simulink library "embdlinuxlib"  (R2018b)
settings: Solver=ode45  StartTime=0.0  StopTime=10.0  RelTol=1e-3
undefined symbols (not defined in the file or in its folder): gcbh, hw, realtime
settings Model: FPTRunName=Active  ModifiedByFormat=The MathWorks Inc.  Creator=The MathWorks, Inc.  LastModifiedBy=The MathWorks Inc.
settings DataIOCC: LimitDataPoints=on  SaveFormat=Array  SignalLoggingSaveFormat=ModelDataLogs
settings OptimizationCC: BlockReduction=off  BooleanDataType=off  ExpressionDepthLimit=2147483647  LifeSpan=inf
settings DebuggingCC: SaveWithParameterizedLinksMsg=none  UnderspecifiedInitializationDetection=Classic  MergeDetectMultiDrivingBlocksExec=none  SignalResolutionControl=TryResolveAllWithWarning  FcnCallInpInsideContextMsg=warning  AllowSymbolicDim=off  StateNameClashWarn=warning  LibraryContextMissingDiagnostic=none  SFUnexpectedBacktrackingDiag=warning  SFNoUnconditionalDefaultTransitionDiag=warning  SFExecutionAtInitializationDiag=none
settings HardwareCC: ProdBitPerPointer=32  ProdBitPerSizeT=32  ProdBitPerPtrDiffT=32  ProdLargestAtomicFloat=None  ProdIntDivRoundTo=Undefined  ProdEndianess=Unspecified  ProdWordSize=32  ProdHWDeviceType=32-bit Generic  TargetUnknown=on
settings ModelReferenceCC: PropagateSignalLabelsOutOfModel=off
settings SFSimCC: SimUseLocalCustomCode=off
settings RTWCC: RTWUseLocalCustomCode=off
settings CodeAppCC: StateflowObjectComments=on
settings GRTTargetCC: TargetLangStandard=C89/C90 (ANSI)  GeneratePreprocessorConditionals=Disable all  CombineOutputUpdateFcns=off  GRTInterface=on
settings ConfigComp: CovMetricSettings=dw  CovHtmlReporting=on  CovSaveCumulativeToWorkspaceVar=on  CovSaveSingleToWorkspaceVar=on  CovShowResultsExplorer=off  CovExternalEMLEnable=off  CovSFcnEnable=off

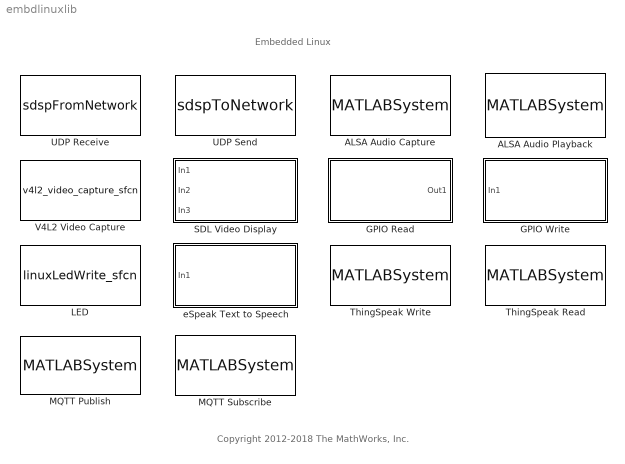
== system embdlinuxlib ==
  note: Copyright 2012-2018 The MathWorks, Inc.
  note: Embedded Linux
  ALSA Audio Capture : MATLABSystem  InitFcn=realtime.internal.ALSAAudioCaptureCallback(gcbh)  System=codertarget.linux.blocks.ALSAAudioCapture  deviceStr=hw:1,0  DataBitDepth=16-bit integer  numberOfChannels=numberOfChannels  sampleRateEnum=sampleRateEnum  frameSize=frameSize  QueueDuration=QueueDuration  blockPlatform=RASPBERRYPI  mask(codertarget.linux.blocks.ALSAAudioCapture){deviceStr=hw:1,0, DataBitDepth=16-bit integer, numberOfChannels=2, sampleRateEnum=44100, frameSize=4410, QueueDuration=0.5, blockPlatform=RASPBERRYPI}
      mask prompts: deviceStr "Device name:"; DataBitDepth "Device Bit depth:"; numberOfChannels "Number of channels(C):"; sampleRateEnum "Audio sampling frequency (Hz):"; frameSize "Samples per frame(N):"; QueueDuration "Queue duration (seconds):"; blockPlatform "Block platform:"
      mask help:
      | Captures audio from the sound card using ALSA driver framework.
      |
      | The block outputs audio data as NxC array, where N is the samples per audio channel and C is the number of chanels.
      |
      | Enter the device name and the number of channels supported by the device. Use the Audio sampling frequency parameter to set the sampling rate in Hertz(Hz). Sample time of the block will be derived from the sampling frequency and the Samples per frame(N) specified by the user.
      mask TypeOptions deviceStr: deviceStr
      mask TypeOptions DataBitDepth: DataBitDepth
      mask TypeOptions numberOfChannels: numberOfChannels
      mask TypeOptions sampleRateEnum: sampleRateEnum
      mask TypeOptions frameSize: frameSize
      mask TypeOptions QueueDuration: QueueDuration
      mask TypeOptions blockPlatform: blockPlatform
      mask Display:
      | color('white');
      | 
      | plot([100,100,100,100],[100,100,100,100]);
      | 
      | plot([0,0,0,0],[0,0,0,0]);
      | 
      | color('black');
      | 
      | text(50, 12,'Device: hw:1,0', 'horizontalAlignment','center','verticalAlignment','middle');
      | 
      | color('blue');
      | 
      | text(96, 90, 'RASPBERRYPI', 'horizontalAlignment', 'right');
      | 
      | color('black');
      | 
      | image('sound_sensor.gif','center');
  ALSA Audio Playback : MATLABSystem  System=codertarget.linux.blocks.ALSAAudioPlayback  deviceStr=hw:0,0  sampleRateEnum=sampleRateEnum  queueDuration=queueDuration  blockPlatform=RASPBERRYPI  mask(codertarget.linux.blocks.ALSAAudioPlayback){deviceStr=hw:0,0, sampleRateEnum=44100, queueDuration=0.5, blockPlatform=RASPBERRYPI}
      mask prompts: deviceStr "Device name:"; sampleRateEnum "Audio sampling frequency (Hz):"; queueDuration "Queue duration (seconds):"; blockPlatform "Block platform:"
      mask help:
      | Sends audio to the sound card for playback using ALSA driver framework.
      |
      | The block accepts NxC array of type int8, int16 or int32, where N is the samples per audio channel and C is the number of channels.
      |
      | Enter the device name and use the Audio sampling frequency parameter to set the sampling rate in Hertz (Hz).
      mask TypeOptions deviceStr: deviceStr
      mask TypeOptions sampleRateEnum: sampleRateEnum
      mask TypeOptions queueDuration: queueDuration
      mask TypeOptions blockPlatform: blockPlatform
      mask Display:
      | color('white');
      | 
      | plot([100,100,100,100],[100,100,100,100]);
      | 
      | plot([0,0,0,0],[0,0,0,0]);
      | 
      | color('black');
      | 
      | text(50, 12,'Device: hw:0,0', 'horizontalAlignment','center','verticalAlignment','middle');
      | 
      | color('blue');
      | 
      | text(96, 90, 'RASPBERRYPI', 'horizontalAlignment', 'right');
      | 
      | color('black');
      | 
      | image('speaker.gif','center');
  GPIO Read : Subsystem  DialogController=linuxDDGCreate  InitFcn=|  mask(GPIO Read){board=Model B+, gpio=17, internalResistor=Off, sampleTime=0.1, direction=Input, blockPlatform=Raspberry Pi}
      | realtime.internal.validateLinuxBlock(get_param(gcbh,'blockPlatform'), gcbh);
      | realtime.internal.gpioCheckParameters(gcs,gcb);
      | realtime.internal.validateGPIO(gcb);
      mask prompts: gpio "GPIO number:"; internalResistor "Internal resistor:"; sampleTime "Sample time:"; blockPlatform "Block platform:"
      mask help: Reads the logical value of a specified GPIO pin configured as input. Select the GPIO input number. Select the internal resistor. Use only one block per GPIO.
      mask init:
      | h = realtime.internal.BoardInfo(blockPlatform);
      | pinName = h.getGPIOPrimaryFunction(board, gpio);
      | pinName = uint8([pinName, 0]); % Add C string termination character
      | switch (internalResistor)
      |     case {'Off'}
      |         resistor = 1;
      |     case {'Pull-up'}
      |         resistor = 2;
      |     case {'Pull-down'}
      |         resistor = 3;
      |     otherwise
      |         resistor = 255; %N/A
      | end
      | realtime.internal.linuxGpioRead('MaskInitialization');
      mask Help: eval('realtime.helpView(get_param(gcb, ''blockPlatform''), [realtime.internal.getHelpLinkPrefix(gcb) ''libgpioread''])');
      mask TypeOptions direction: Input | Output
      mask Display:
      | text(0.5, 0.15, 'GPIO 17', 'horizontalAlignment', 'center');
      | image(imread('digitalio.png'),[0.32 0.25 0.35 0.55]);
      | color('blue');
      | text(0.90, 0.90, 'RASPBERRYPI', 'horizontalAlignment', 'right');
      | color('black');
  GPIO Write : Subsystem  DialogController=linuxDDGCreate  InitFcn=|  mask(GPIO Write){board=Model B+, gpio=4, direction=Output, blockPlatform=Raspberry Pi}
      | realtime.internal.validateLinuxBlock(get_param(gcbh,'blockPlatform'), gcbh);
      | realtime.internal.gpioCheckParameters(gcs,gcb);
      | realtime.internal.validateGPIO(gcb);
      mask prompts: gpio "GPIO number:"; blockPlatform "Block platform:"
      mask help: Sets the logical value of a GPIO pin configured as output. Select the GPIO output number. Do not assign the same GPIO number to multiple blocks within a model.
      mask init:
      | h = realtime.internal.BoardInfo(blockPlatform);
      | realtime.internal.linuxGpioWrite('MaskInitialization');
      mask Help: eval('realtime.helpView(get_param(gcb, ''blockPlatform''), [realtime.internal.getHelpLinkPrefix(gcb) ''libgpiowrite''])');
      mask TypeOptions direction: Input | Output
      mask Display:
      | text(0.5, 0.15, 'GPIO 4', 'horizontalAlignment', 'center');
      | image(imread('digitalio.png'),[0.32 0.25 0.35 0.55]);
      | color('blue');
      | text(0.90, 0.90, 'RASPBERRYPI', 'horizontalAlignment', 'right');
      | color('black');
  LED : S-Function  DialogController=linuxDDGCreate  InitFcn=realtime.internal.validateLinuxBlock(get_param(gcbh, 'blockPlatform'), gcbh);  FunctionName=linuxLedWrite_sfcn  Parameters=deviceFile  SFunctionDeploymentMode=off  EnableBusSupport=off  mask(LED Write){board=BeagleBoard xM, led=PMU_STAT (Green), blockPlatform=Raspberry Pi}
      mask prompts: blockPlatform "Block platform:"
      mask help:
      | Turns an LED on or off.
      |
      | Select the desired LED from the drop down menu. Do not use the same LED
      | in multiple blocks within a model.
      mask init:
      | hBoard = realtime.internal.BoardInfo(blockPlatform);
      | deviceFile = hBoard.getLEDDeviceFile(board, led);
      | deviceFile = uint8([deviceFile, 0]);
      | realtime.internal.linuxLedWrite('MaskInitialization');
      mask Help: eval('realtime.helpView(get_param(gcb, ''blockPlatform''),[realtime.internal.getHelpLinkPrefix(gcb) ''libled''])');
      mask Display:
      | text(0.5, 0.15, 'PMU_STAT (Green)', 'horizontalAlignment', 'center');
      | image(imread('led.png'),[0.32 0.25 0.35 0.55]);
      | color('blue');
      | text(0.90, 0.90, 'RASPBERRYPI', 'horizontalAlignment', 'right');
      | color('black');
  MQTT Publish : MATLABSystem  System=codertarget.linux.blocks.MQTTPublish  Topic=topic/level  QoS=0  RetainMsg=off
      mask Type: codertarget.linux.blocks.MQTTPublish
      mask Display:
      | color('white');
      | 
      | plot([100,100,100,100],[100,100,100,100]);
      | 
      | plot([0,0,0,0],[0,0,0,0]);
      | 
      | color('black');
      | 
      | port_label('input',1,'Msg');
      | 
      | port_label('output',1,'Status');
      | 
      | text(50, 12,'topic/level', 'horizontalAlignment','center','verticalAlignment','middle');
      | 
      | color('blue');
      | 
      | text(96, 90, 'RASPBERRYPI', 'horizontalAlignment', 'right');
  MQTT Subscribe : MATLABSystem  System=codertarget.linux.blocks.MQTTSubscribe  Topic=topic/level/#  QoS=0  MessageLength=1  SampleTime=1
      mask Type: codertarget.linux.blocks.MQTTSubscribe
      mask Display:
      | color('white');
      | 
      | plot([100,100,100,100],[100,100,100,100]);
      | 
      | plot([0,0,0,0],[0,0,0,0]);
      | 
      | color('black');
      | 
      | port_label('output',1,'IsNew');
      | 
      | port_label('output',3,'Topic');
      | 
      | port_label('output',2,'Msg');
      | 
      | text(50, 12,'topic/level/#', 'horizontalAlignment','center','verticalAlignment','middle');
      | 
      | color('blue');
      | 
      | text(96, 90, 'RASPBERRYPI', 'horizontalAlignment', 'right');
      | 
      | color('black');
  SDL Video Display : Subsystem  InitFcn=|  TreatAsAtomicUnit=on  mask(SDL Video Display){pixelFormat=RGB, pixelOrder=Planar, rowMajor=on, blockPlatform=Raspberry Pi}
      | realtime.internal.validateLinuxBlock(get_param(gcbh,'blockPlatform'),gcbh);
      | realtime.internal.sdl_video_display_callback('BlockCheck',gcbh);
      mask prompts: pixelFormat "Pixel format:"; pixelOrder "Pixel order:"; rowMajor "Input image is transposed (data is row major)"; blockPlatform "Block platform:"
      mask help: Displays video using Simple Directmedia Layer (SDL) multimedia library. Use Pixel format parameter to specify the format of the input video stream. Only one SDL Video Display block is allowed in a Simulink model.
      mask init:
      | realtime.internal.sdl_video_display_callback('MaskInitialization',gcbh);
      mask Help: eval('realtime.helpView(get_param(gcb, ''blockPlatform''),[realtime.internal.getHelpLinkPrefix(gcb) ''libsdlvideodisplay''])');
      mask TypeOptions pixelFormat: RGB | YCbCr 4:2:2
      mask TypeOptions pixelOrder: Planar | Interleaved
      mask Display:
      | color('blue');
      | text(0.90, 0.90, 'RASPBERRYPI', 'horizontalAlignment', 'right');
      | color('black');
      | [data, map]=imread('LCD.gif');pic=ind2rgb(data,map);image(pic,[0.32 0.25 0.35 0.55]);
      | port_label('input', 1, 'R');
      | port_label('input', 2, 'G');
      | port_label('input', 3, 'B');
  ThingSpeak Read : MATLABSystem  System=codertarget.linux.blocks.ThingSpeakRead  ChannelID=12345  ChannelAccess=Public  ReadAPIKey=ABCDEFGHIJK  FieldNumber=1  PrintDiagnosticMessages=off  SampleTime=60
      mask Type: codertarget.linux.blocks.ThingSpeakRead
      mask Display:
      | color('white');
      | 
      | plot([100,100,100,100],[100,100,100,100]);
      | 
      | plot([0,0,0,0],[0,0,0,0]);
      | 
      | color('black');
      | 
      | port_label('output',1,'Field1');
      | 
      | port_label('output',2,'Status');
      | 
      | text(50, 12,'Channel:12345', 'horizontalAlignment','center','verticalAlignment','middle');
      | 
      | color('blue');
      | 
      | text(96, 90, 'RASPBERRYPI', 'horizontalAlignment', 'right');
      | 
      | color('black');
      | 
      | image('cloudread_linux.png','center');
  ThingSpeak Write : MATLABSystem  InitFcn=realtime.internal.validateLinuxBlock(get_param(gcbh, 'blockPlatform'), gcbh);  System=codertarget.linux.blocks.ThingSpeakWrite  UpdateURL=https://api.thingspeak.com/update  WriteAPIKey=<Enter the write API key for your channel>  NumberOfVariables=1  UpdateInterval=UpdateInterval  PrintDiagnosticMessages=off  CoordinatesEnabled=off  CoordinatesSource=Block dialog  Coordinates=Coordinates  StatusEnabled=off  StatusSource=Block dialog  StatusMessage=OK  mask(codertarget.linux.blocks.ThingSpeakWrite){UpdateURL=https://api.thingspeak.com/update, WriteAPIKey=<Enter the write API key for your channel>, NumberOfFields=1, UpdateInterval=60, PrintDiagnosticMessages=off, CoordinatesEnabled=off, CoordSrc=Block dialog, Coordinates=[42.29971, -71.350719, 69.29], blockPlatform=Raspberry Pi}
      mask prompts: UpdateURL "Update URL:"; WriteAPIKey "Write API key:"; NumberOfFields "Number of variables to send:"; UpdateInterval "Update interval:"; PrintDiagnosticMessages "Print diagnostic messages"; CoordinatesEnabled "Send location information"; CoordSrc "Coordinate source:"; Coordinates "Coordinates (latitude, longitude, altitude):"; blockPlatform "Block platform:"
      mask help:
      | Send data to ThingSpeak, MathWorks IoT Analytics Platform.
      | The hardware must be connected to the Internet. Input ports only accept numeric scalar signals.
      |
      | Enter the Write API Key for your ThingSpeak channel. Each input variable is written to a field in your ThingSpeak channel.
      | Set Update interval to the number of seconds to wait between two successive data send requests. Visit your ThingSpeak account page to find the minimum update interval for your channel.
      |
      | Check “Print diagnostic messages” to send the ThingSpeak server response to standard output on the hardware.
      mask init:
      | codertarget.linux.blocks.ThingSpeakWriteCallback('MaskInitialization',gcbh);
      mask Help: eval('realtime.helpView(get_param(gcb, ''blockPlatform''), [realtime.internal.getHelpLinkPrefix(gcb) ''libthingspeakwrite''])');
      mask TypeOptions UpdateURL: UpdateURL
      mask TypeOptions WriteAPIKey: WriteAPIKey
      mask TypeOptions NumberOfFields: 1 | 2 | 3 | 4 | 5 | 6 | 7 | 8
      mask TypeOptions UpdateInterval: UpdateInterval
      mask TypeOptions PrintDiagnosticMessages: PrintDiagnosticMessages
      mask TypeOptions CoordinatesEnabled: CoordinatesEnabled
      mask Callback CoordinatesEnabled: codertarget.linux.blocks.ThingSpeakWriteCallback('CoordinatesEnabled',gcbh);
      mask TypeOptions CoordSrc: Block dialog | Input port
      mask Callback CoordSrc: codertarget.linux.blocks.ThingSpeakWriteCallback('CoordinatesSource',gcbh);
      mask TypeOptions Coordinates: Coordinates
      mask DialogControl DescGroupVar Prompt: ThingSpeak Write
      mask DialogControl Container2 Prompt: Main
      mask DialogControl Container10 Prompt: Optional
      mask Display:
      | image(imread('cloud.png'),[0.25 0.25 0.55 0.45]);
      | color('blue');
      | text(0.35, 0.87, 'RASPBERRYPI', 'horizontalAlignment', 'left');
      | color('black');
      | CoordinatesEnabled = get_param(gcb, 'CoordinatesEnabled');
      | CoordinatesSource = get_param(gcb, 'CoordinatesSource');
      | NumberOfFields_ = str2double(get_param(gcb,'NumberOfFields'));
      | if NumberOfFields_ >= 2
      | port_label('input', 1, 'var1');
      | port_label('input', 2, 'var2');
      | end
      | if NumberOfFields_ >= 3
      | port_label('input', 3, 'var3');
      | end
      | if NumberOfFields_ >= 4
      | port_label('input', 4, 'var4');
      | end
      | if NumberOfFields_ >= 5
      | port_label('input', 5, 'var5');
      | end
      | if NumberOfFields_ >= 6
      | port_label('input', 6, 'var6');
      | end
      | if NumberOfFields_ >= 7
      | port_label('input', 7, 'var7');
      | end
      | if NumberOfFields_ >= 8
      | port_label('input', 8, 'var8');
      | end
      | if strcmp(CoordinatesEnabled, 'on') && strcmp(CoordinatesSource, 'Input port')
      | port_label('input', NumberOfFields_+1, 'location');
      | end
  UDP Receive : S-Function  InitFcn=realtime.internal.validateLinuxBlock(get_param(gcbh, 'blockPlatform'), gcbh);  FunctionName=sdspFromNetwork  Parameters=localURL, localPort, remoteURL, remotePort, recvBufferSize, signalDatatype, dims, sampletime, isVarSize, blockingTime  SFunctionDeploymentMode=off  EnableBusSupport=off  mask(UDP Receive){localURL='0.0.0.0', localPort=25000, remoteURL='0.0.0.0', remotePort=-1, recvBufferSize=8192, signalDatatype=uint8, dims=255, isVarSize=off, showBlockingTime=off, blockingTime=0, sampletime=0.01, blockPlatform=Raspberry Pi}
      mask prompts: localURL "Local IP address:"; localPort "Local IP port:"; remoteURL "Remote IP address ('0.0.0.0' to accept all):"; remotePort "Remote IP port:"; recvBufferSize "Receive buffer size (bytes):"; signalDatatype "Data type:"; dims "Data size (elements):"; isVarSize "Output variable-size signal"; showBlockingTime "Show blocking time"; blockingTime "Blocking time (seconds):"; sampletime "Sample time (seconds):"; blockPlatform "Block Platform"
      mask help:
      | Receives UDP packets from another UDP host on an Internet network. The sending UDP host must send UDP packets to the Local IP port specified in the block mask.
      |
      | Match the Data type parameter with the data type of the incoming data. Match the Data size parameter with the number of elements of the incoming data.
      |
      | For example, if the data type of the incoming data is single and the dimensions are [3x1], set the Data type parameter to single and set the Data size parameter to 3.
      mask init:
      | icon = '';
      | %icon = sprintf('%s\n', 'fprintf(''UDP Receive'');');
      | % If there are multiple ports, label them
      | if strcmp(get_param(gcb,'isVarSize'), 'off')
      |     icon = sprintf('%s%s\n', icon, 'port_label(''output'', 1, ''Data'');');
      |     icon = sprintf('%s%s\n', icon, 'port_label(''output'', 2, ''Size'');');
      | end
      | icon = [icon sprintf('%s\n','color(''blue'');')];
      | icon = [icon '[data, map]=imread(''ethernet1_bw.gif'');pic=ind2rgb(data,map);image(pic,[0.32 0.25 0.40 0.45]);'];
      | platform = realtime.internal.getBlockDisplayText(gcb);
      | icon = [icon sprintf('%s\n',['text(0.97, 0.87, ''' platform ''', ''horizontalalignment'', ''right'');'])];
      | set_param(gcb, 'maskDisplay', icon);
      | 
      | % Hide the lengthDatatype and BlockingTime if required
      | vis = get_param(gcbh, 'MaskVisibilities');
      | vis{10} = get_param(gcbh, 'showBlockingTime');
      | set_param(gcbh, 'MaskVisibilities', vis);
      mask Help: eval('realtime.helpView(get_param(gcb, ''blockPlatform''), [realtime.internal.getHelpLinkPrefix(gcb) ''libudpreceive''])');
      mask TypeOptions signalDatatype: double | single | int8 | uint8 | int16 | uint16 | int32 | uint32 | boolean
      mask Display:
      | port_label('output', 1, 'Data');
      | port_label('output', 2, 'Size');
      | color('blue');
      | [data, map]=imread('ethernet1_bw.gif');pic=ind2rgb(data,map);image(pic,[0.32 0.25 0.40 0.45]);text(0.97, 0.87, 'RASPBERRYPI', 'horizontalalignment', 'right');
  UDP Send : S-Function  InitFcn=realtime.internal.validateLinuxBlock(get_param(gcbh, 'blockPlatform'), gcbh);  FunctionName=sdspToNetwork  Parameters=localURL, localPortSource, localPort, remoteURL, remotePort, separateLengthPort, []  SFunctionDeploymentMode=off  EnableBusSupport=off  mask(UDP Send){remoteURL='255.255.255.255', remotePort=25000, localURL='0.0.0.0', localPortSource=Automatically determine, localPort=-1, sampletime=-1, blockPlatform=Raspberry Pi, separateLengthPort=0}
      mask prompts: remoteURL "Remote IP address ('255.255.255.255' for broadcast):"; remotePort "Remote IP port:"; localURL "Local IP address:"; localPortSource "Local IP port source:"; localPort "Local IP port:"; blockPlatform "Block Platform"; separateLengthPort "Use a separate length port"
      mask help: Sends UDP packets to another UDP host on an Internet network. Set Remote IP address parameter to the IP address of the receiving UDP host. Set the Remote IP port parameter to the port number used by the receiving UDP host.
      mask Help: eval('realtime.helpView(get_param(gcb, ''blockPlatform''), [realtime.internal.getHelpLinkPrefix(gcb) ''libudpsend''])');
      mask TypeOptions localPortSource: Automatically determine | Specify via dialog
      mask Callback localPortSource:
      | mask_vis = get_param(gcbh, 'MaskVisibilities');
      | if strcmp(get_param(gcbh,'localPortSource'),'Specify via dialog')
      |     mask_vis{5} = 'on';
      | else
      |     mask_vis{5} = 'off';
      | end
      | set_param(gcbh, 'MaskVisibilities', mask_vis);
      | clear('mask_vis');
      mask Display:
      | %fprintf('UDP Send');
      | color('blue');
      | [data, map]=imread('ethernet2_bw.gif');pic=ind2rgb(data,map);image(pic,[0.32 0.25 0.40 0.45]);
      | platform = realtime.internal.getBlockDisplayText(gcb);
      | text(0.97, 0.87, platform, 'horizontalalignment', 'right');
  V4L2 Video Capture : S-Function  InitFcn=realtime.internal.validateLinuxBlock(get_param(gcbh, 'blockPlatform'), gcbh);  FunctionName=v4l2_video_capture_sfcn  Parameters=devName, roiTop, roiLeft, roiWidth, roiHeight, width, height, pixelFormat, pixelOrder, simOutput, sampleTime  SFunctionModules=v4l2_capture  SFunctionDeploymentMode=off  EnableBusSupport=off  mask(V4L2 Video Capture){m_devName='/dev/video0', roi=[0, 0, 640, 480], imSizeSelection=320x240, imSize=[640, 480], pixelFormat=RGB, pixelOrder=Planar, sampleTime=1/10, simOutput=Colorbars, blockPlatform=Raspberry Pi}
      mask prompts: m_devName "Device name:"; roi "Region of interest ([top, left, width, height]):"; imSizeSelection "Image size:"; imSize "Image size ([width, height]):"; pixelFormat "Pixel format:"; pixelOrder "Pixel order:"; sampleTime "Sample time:"; simOutput "Simulation output:"; blockPlatform "Block platform:"
      mask help:
      | Captures video from a USB camera using V4L2 driver framework. During simulation, the model outputs a moving colorbar image. While running on hardware, the block outputs video from a USB camera.
      |
      | Set Image size parameter to the desired output size. Use Pixel format parameter to specify the format of the output video stream.
      mask init:
      | [devName, roiTop, roiLeft, roiWidth, roiHeight, width, height] = realtime.internal.v4l2Setup(m_devName, roi, imSizeSelection, imSize, pixelFormat, simOutput);
      | realtime.internal.v4l2_video_capture_callback('MaskInitialization');
      mask Help: eval('realtime.helpView(get_param(gcb, ''blockPlatform''),[realtime.internal.getHelpLinkPrefix(gcb) ''libv4l2videocapture''])');
      mask TypeOptions imSizeSelection: 160x120 | 320x240 | 640x480 | 800x600 | Custom
      mask Callback imSizeSelection: realtime.internal.v4l2_video_capture_callback('imSizeSelection');
      mask TypeOptions pixelFormat: YCbCr 4:2:2 | RGB
      mask TypeOptions pixelOrder: Interleaved | Planar
      mask TypeOptions simOutput: Colorbars | Black | White | Live video from camera (Linux host only)
      mask Display:
      | color('blue');
      | text(0.90, 0.90, 'RASPBERRYPI', 'horizontalAlignment', 'right');
      | color('black');
      | pic=imread('webcam.png');image(pic,[0.32 0.25 0.35 0.55]);port_label('output', 1, 'R');
      | port_label('output', 2, 'G');
      | port_label('output', 3, 'B');
  eSpeak Text to Speech : Subsystem  InitFcn=realtime.internal.validateLinuxBlock(get_param(gcbh, 'blockPlatform'), gcbh);  mask(eSpeak Text to Speech){blockPlatform=Raspberry Pi}
      mask prompts: blockPlatform "Block platform:"
      mask help:
      | Converts text to speech using eSpeak speech synthesizer. The synthesized speech is output by the default audio device.
      |
      | The input port accepts a uint8 array containing the ASCII text to be converted.
      mask init:
      | realtime.internal.linuxTexttospeech('MaskInitialization');
      mask Help: eval('realtime.helpView(get_param(gcb, ''blockPlatform''), [realtime.internal.getHelpLinkPrefix(gcb) ''libespeaktexttospeech''])');
      mask Display:
      | image(imread('text_to_speech.png'),[0.32 0.25 0.35 0.55]);
      | color('blue');
      | text(0.90, 0.90, 'RASPBERRYPI', 'horizontalAlignment', 'right');
      | color('black');

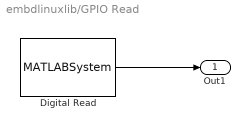
== system embdlinuxlib/GPIO Read ==
  Digital Read : MATLABSystem  System=codertarget.linux.blocks.DigitalRead  PinNumber=gpio  SampleTime=sampleTime
      mask Type: codertarget.linux.blocks.DigitalRead
      mask Display:
      | disp('Digital Read');
      | port_label('output',1,'y');
  Out1 : Outport
  wires:
  Digital Read/1 -> Out1/1

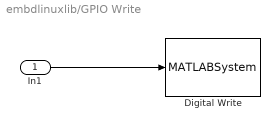
== system embdlinuxlib/GPIO Write ==
  In1 : Inport
  Digital Write : MATLABSystem  System=codertarget.linux.blocks.DigitalWrite  PinNumber=gpio
      mask Type: codertarget.linux.blocks.DigitalWrite
      mask Display:
      | disp('Digital Write');
      | port_label('input',1,'u');
  wires:
  In1/1 -> Digital Write/1

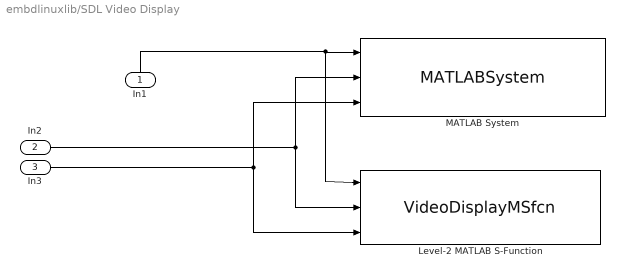
== system embdlinuxlib/SDL Video Display ==
  In1 : Inport
  In2 : Inport  Port=2
  In3 : Inport  Port=3
  Level-2 MATLAB S-Function : M-S-Function  FunctionName=VideoDisplayMSfcn  Parameters=pixelFormat
      settings: DeleteFcn=realtime.internal.sdl_video_display_callback('Close',gcbh);  ModelCloseFcn=realtime.internal.sdl_video_display_callback('Close',gcbh);
  MATLAB System : MATLABSystem  System=codertarget.linux.blocks.SDLVideoDisplay  PixelFormat=RGB
      mask Type: codertarget.linux.blocks.SDLVideoDisplay
      mask Display:
      | disp('SDLVideoDisplay');
      | port_label('input',1,'pln1');
      | port_label('input',2,'pln2');
      | port_label('input',3,'pln3');
  wires:
  In3/1 -> MATLAB System/3, Level-2 MATLAB S-Function/3
  In2/1 -> MATLAB System/2, Level-2 MATLAB S-Function/2
  In1/1 -> MATLAB System/1, Level-2 MATLAB S-Function/1

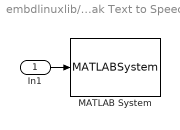
== system embdlinuxlib/eSpeak Text to Speech ==
  In1 : Inport
  MATLAB System : MATLABSystem  System=codertarget.linux.blocks.Espeak  Pitch=50  Options=""
      mask Type: codertarget.linux.blocks.Espeak
      mask Display:
      | disp('Espeak');
      | port_label('input',1,'u');
  wires:
  In1/1 -> MATLAB System/1
